simulink model "three"  (R2020b)
settings: Solver=VariableStepAuto  StartTime=0.0  StopTime=10.0  RelTol=1e-3
values from neighbouring files (symbols this model uses):
  b = 50.0    [variable.sldd]
  Ki = 50.0    [threeParameters.sldd]    (also in variable.sldd)
  Kp = 600.0    [threeParameters.sldd]    (also in variable.sldd)
  m = 1000.0    [variable.sldd]
settings Model: Creator=USER  LastModifiedBy=USER

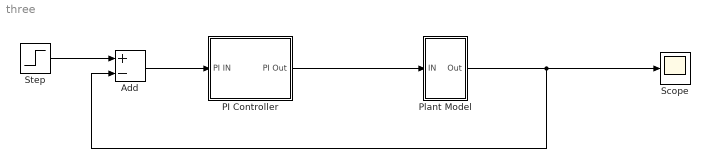
== system three ==
  Add : Sum  Inputs=+-
  PI Controller : Subsystem
  Plant Model : Subsystem
  Scope : Scope
  Step : Step  SampleTime=0
  wires:
  PI Controller/1(PI Out) -> Plant Model/1(IN)
  Plant Model/1(Out) -> Add/2, Scope/1
  Step/1 -> Add/1
  Add/1 -> PI Controller/1(PI IN)

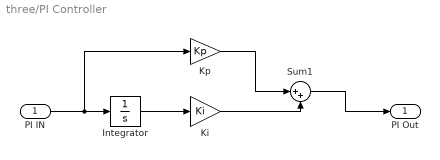
== system three/PI Controller ==
  PI IN : Inport  OutDataTypeStr=double  PortDimensions=1  SampleTime=0
  Integrator : Integrator
  Ki : Gain  Gain=Ki
  Kp : Gain  Gain=Kp
  Sum1 : Sum  Inputs=|++
  PI Out : Outport  OutDataTypeStr=double  PortDimensions=1  SampleTime=0
  wires:
  Ki/1 -> Sum1/2
  PI IN/1 -> Integrator/1, Kp/1
  Kp/1 -> Sum1/1
  Sum1/1 -> PI Out/1
  Integrator/1 -> Ki/1

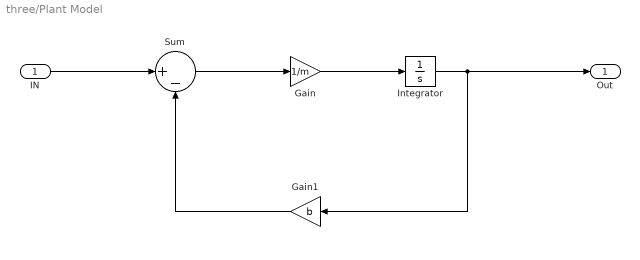
== system three/Plant Model ==
  IN : Inport
  Gain : Gain  Gain=1/m
  Gain1 : Gain  Gain=b
  Integrator : Integrator
  Sum : Sum  Inputs=|+-
  Out : Outport
  wires:
  Gain1/1 -> Sum/2
  Sum/1 -> Gain/1
  IN/1 -> Sum/1
  Gain/1 -> Integrator/1
  Integrator/1 -> Out/1, Gain1/1
